simulink model "test_lpvanalysis_mdl"  (R2018b)
settings: Solver=VariableStepAuto  StartTime=0.0  StopTime=100  MaxStep=0.01  RelTol=1e-3  EnableMultiTasking=on
libraries: lpvlibrary x1
settings Model: Creator=Fernando  LastModifiedBy=ferna
settings OptimizationCC: LifeSpan=inf
settings DebuggingCC: SFUnexpectedBacktrackingDiag=warning  SFNoUnconditionalDefaultTransitionDiag=warning
settings SFSimCC: SimUseLocalCustomCode=off
settings RTWCC: RTWUseLocalCustomCode=off
settings CodeAppCC: StateflowObjectComments=on
settings GRTTargetCC: TargetLangStandard=C89/C90 (ANSI)  GeneratePreprocessorConditionals=Disable all
settings ConfigComp: CovMetricSettings=dw  CovHtmlReporting=on  CovSaveCumulativeToWorkspaceVar=on  CovSaveSingleToWorkspaceVar=on  CovExternalEMLEnable=off

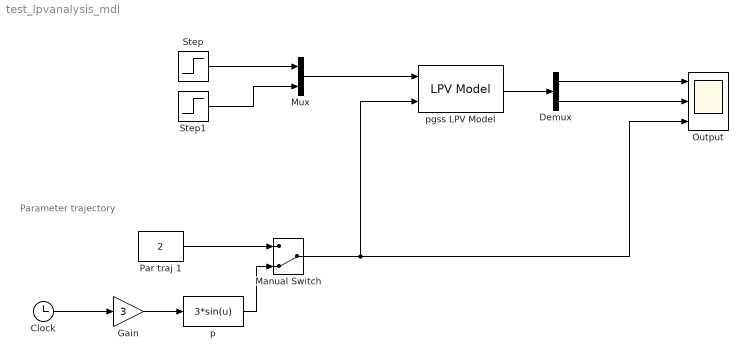
== system test_lpvanalysis_mdl ==
  note: Parameter trajectory
  Clock : Clock
  Demux : Demux  Outputs=2
  Gain : Gain  Gain=3
  Manual Switch : ManualSwitch  CurrentSetting=0
  Mux : Mux  Inputs=2
  Output : Scope  NumInputPorts=3
  Par traj 1 : Constant  Value=2
  Step : Step  Time=0.2  SampleTime=0
  Step1 : Step  Time=0.2  SampleTime=0
  p : Fcn  Expr=3*sin(u)
  pgss LPV Model : lpvlibrary/LPV Model  pdG=pdG  x0=0
      settings: SourceProductName=LPV Toolbox
  wires:
  Clock/1 -> Gain/1
  p/1 -> Manual Switch/2
  Par traj 1/1 -> Manual Switch/1
  Manual Switch/1 -> Output/3, pgss LPV Model/2
  Demux/1 -> Output/1
  Step/1 -> Mux/1
  Step1/1 -> Mux/2
  Mux/1 -> pgss LPV Model/1
  pgss LPV Model/1 -> Demux/1
  Demux/2 -> Output/2
  Gain/1 -> p/1
